simulink model "untitled"  (R2021b)
settings: Solver=VariableStepAuto  StartTime=0.0  StopTime=10.0  RelTol=1e-3
values from neighbouring files (symbols this model uses):
  simu = simulationClass()    [wecSimInputFile.m]
undefined symbols (not defined in the file or in its folder): DiscIntNeverNeededParam, PTOSimBlock
settings Model: Creator=jleonqu  LastModifiedBy=jleonqu

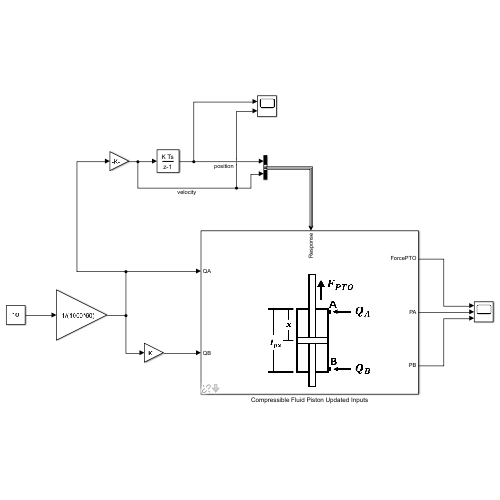
[thumbnail: Simulink's stored preview of the top-level diagram]
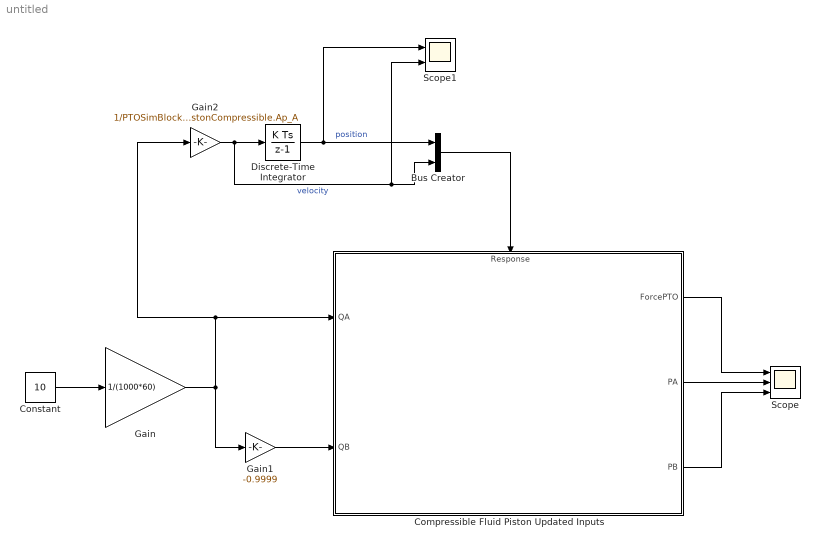
== system untitled ==
  Bus Creator : BusCreator  Inputs=2
  Compressible Fluid Piston Updated Inputs : Subsystem  AncestorBlock=PTOSim_Lib_UpdatedV3/Hydraulic/Compressible Fluid Piston Updated Inputs  mask{PTOSimBlock=PTOSimBlock(1), InputFileText=Use WEC-Sim input file to define PTO parameters, Ap_A=0, Ap_B=0, PistonStroke=0, BulkModulus=0, xi_piston=0, pAi=0, pBi=0}
      mask prompts: PTOSimBlock "Piston Name"; Ap_A "Piston area A [m]"; Ap_B "Piston area B [m]"; PistonStroke "Piston stroke [m]"; BulkModulus "Fluid Bulk Modulus [Pa]"; xi_piston "Piston initial displacement from A [m]"; pAi "Port A Initial pressure [Pa]"; pBi "Port B Initial pressure [Pa]"
      mask help:
      | PTO-Sim Compressible Fluid Piston
      |
      | This block simualtes a hydraulic cylinder using a compressible fluid model. The block inputs are Response, QA and QB. Response is the signal output of the block Rotational PTO Actuation Force. QA and QB are the flow rate for port A and port B of the cylinder. The outputs of the block are ForcePTO, PA, and PB.
      mask init:
      | if exist('PTOSimBlock','var')
      |     h=[gcb '/To Workspace'];
      |     responseName=['PTOSimBlock' num2str(PTOSimBlock.PTOSimBlockNum) '_out'];
      |     set_param(h,'VariableName',responseName);
      | end
      | clear h responseName
      | %HydraulicBlock.checkLoc('W');
      settings: PortSchema="{\"entries\":[{\"content\":{\"sides\":[{\"content\":{\"connectorIds\":[\"In1\",\"In2\"]},\"type\":\"ConnectorPlacement.EquallySpacedRectSide\",\"uuid\":\"572dbc7c-8f4c-46fc-9000-663c89355fbd\"},{\"content\":{\"connectorIds\":[\"Out1\",\"Out2\",\"Out3\"],\"side\":\"RIGHT\"},\"type\":\"ConnectorPlacement.EquallySpacedRectSide\",\"uuid\":\"3b7821ce-a540-4de1-8f34-0d55375c774c\"},{\"content\":{\"connectorIds\":[\"In3\"],\"side\":\"TOP\"},\"type\":\"ConnectorPlacement.EquallySpacedRectSide\",\"uuid\":\"b6f5c275-868d-447d-b609-cdda14e9f222\"},{\"content\":{\"connectorIds\":[],\"side\":\"HIDDEN\"},\"type\":\"ConnectorPlacement.EquallySpacedRectSide\",\"uuid\":\"5b34aa5d-01fb-4d75-9f22-3e4ce64ee132\"}]},\"type\":\"ConnectorPlacement.EquallySpacedConnector\",\"uuid\":\"5b16a2f7-6624-4a26-89bf-8d87cef610e1\"}],\"packageUris\":[\"http://schema.mathworks.com/mf0/Connector/R2020b\"],\"version\":\"1.0\"}"
      mask Help:
      | This block simualtes a hydraulic cylinder using a compressible fluid model. The block inputs are Response and HydraulicInput. Response is the signal output of the block Rotational PTO Actuation Force. HydraulicInput is a two signal vector with the information of the flow rate for port A and port B of the cylinder. The output of the block is PistonOutput, which is a three signal vector with PressureA, PressureB, and ForcePTO.
      | 
      | The outputs are calculated using the model presented in the following link: http://wec-sim.github.io/WEC-Sim/master/user/advanced_features.html#pto-sim
      mask DialogControl ParameterGroupVar Prompt: Custom Parameters
      mask DialogControl PistonProperties Prompt: Piston Properties
      mask DialogControl InitialConditions Prompt: Initial Conditions
      mask Display: image('DoubleActingPiston.png'); % Use "Edit Image" on toolstrip to change.
  Constant : Constant  Value=10
  Discrete-Time Integrator : DiscreteIntegrator  SampleTime=-1  ICPrevOutput=DiscIntNeverNeededParam  ICPrevScaledInput=DiscIntNeverNeededParam
  Gain : Gain  Gain=1/(1000*60)
  Gain1 : Gain  Gain=-0.9999
  Gain2 : Gain  Gain=1/PTOSimBlock(1).HydPistonCompressible.Ap_A
  Scope : Scope  NumInputPorts=3
  Scope1 : Scope  NumInputPorts=2
  wires:
  Constant/1 -> Gain/1
  Gain1/1 -> Compressible Fluid Piston Updated Inputs/2(QB)
  Gain/1 -> Gain1/1, Compressible Fluid Piston Updated Inputs/1(QA), Gain2/1
  Gain2/1 -> Scope1/2, Bus Creator/2, Discrete-Time Integrator/1  "velocity"
  Discrete-Time Integrator/1 -> Scope1/1, Bus Creator/1  "position"
  Bus Creator/1 -> Compressible Fluid Piston Updated Inputs/3(Response)
  Compressible Fluid Piston Updated Inputs/1(ForcePTO) -> Scope/1
  Compressible Fluid Piston Updated Inputs/2(PA) -> Scope/2
  Compressible Fluid Piston Updated Inputs/3(PB) -> Scope/3

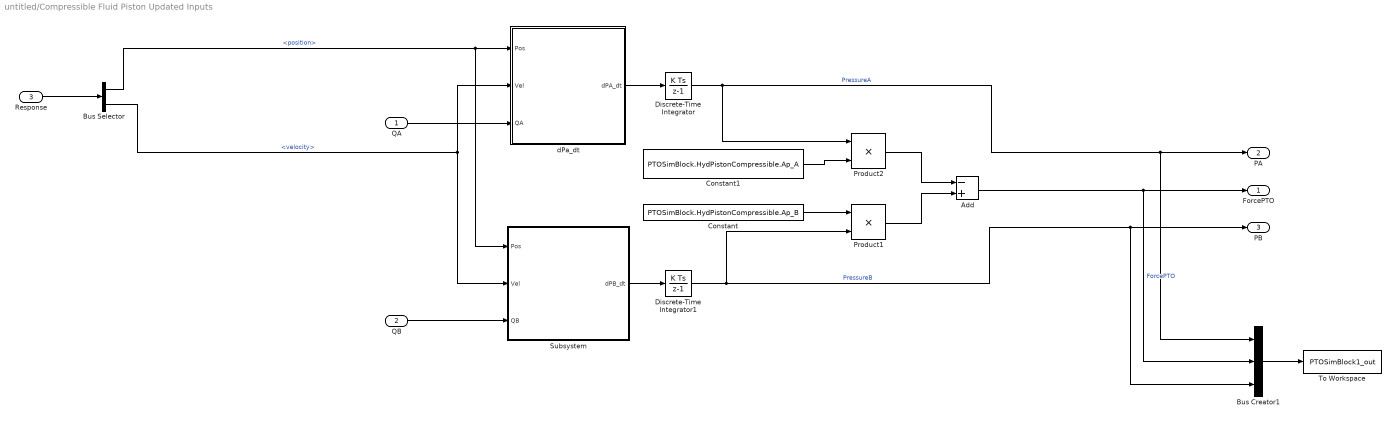
== system untitled/Compressible Fluid Piston Updated Inputs ==
  QA : Inport
  QB : Inport  Port=2
  Response : Inport  Port=3
  Add : Sum  Inputs=-+
  Bus Creator1 : BusCreator  Inputs=3
  Bus Selector : BusSelector  OutputSignals=position,velocity
  Constant : Constant  Value=PTOSimBlock.HydPistonCompressible.Ap_B
  Constant1 : Constant  Value=PTOSimBlock.HydPistonCompressible.Ap_A
  Discrete-Time Integrator : DiscreteIntegrator  InitialCondition=PTOSimBlock.HydPistonCompressible.pAi  SampleTime=-1  ICPrevOutput=DiscIntNeverNeededParam  ICPrevScaledInput=DiscIntNeverNeededParam
  Discrete-Time Integrator1 : DiscreteIntegrator  InitialCondition=PTOSimBlock.HydPistonCompressible.pBi  SampleTime=-1  ICPrevOutput=DiscIntNeverNeededParam  ICPrevScaledInput=DiscIntNeverNeededParam
  Product1 : Product
  Product2 : Product
  Subsystem : Subsystem  AncestorBlock=PTOSim_Lib_UpdatedV3/Hydraulic/Compressible Fluid Piston Updated/Subsystem
  To Workspace : ToWorkspace  VariableName=PTOSimBlock1_out  SaveFormat=Structure With Time  SampleTime=simu.dtOut
  dPa_dt : Subsystem  AncestorBlock=PTOSim_Lib_UpdatedV3/Hydraulic/Compressible Fluid Piston Updated/dPa_dt
  ForcePTO : Outport
  PA : Outport  Port=2
  PB : Outport  Port=3
  wires:
  Bus Selector/1 -> dPa_dt/1(Pos), Subsystem/1(Pos)  "<position>"
  Discrete-Time Integrator/1 -> Product2/1, Bus Creator1/1, PA/1  "PressureA"
  Response/1 -> Bus Selector/1
  Subsystem/1(dPB_dt) -> Discrete-Time Integrator1/1
  Bus Selector/2 -> dPa_dt/2(Vel), Subsystem/2(Vel)  "<velocity>"
  Constant/1 -> Product1/1
  Product2/1 -> Add/1
  dPa_dt/1(dPA_dt) -> Discrete-Time Integrator/1
  Product1/1 -> Add/2
  QB/1 -> Subsystem/3(QB)
  Bus Creator1/1 -> To Workspace/1
  Add/1 -> ForcePTO/1, Bus Creator1/2  "ForcePTO"
  Discrete-Time Integrator1/1 -> Product1/2, PB/1, Bus Creator1/3  "PressureB"
  Constant1/1 -> Product2/2
  QA/1 -> dPa_dt/3(QA)

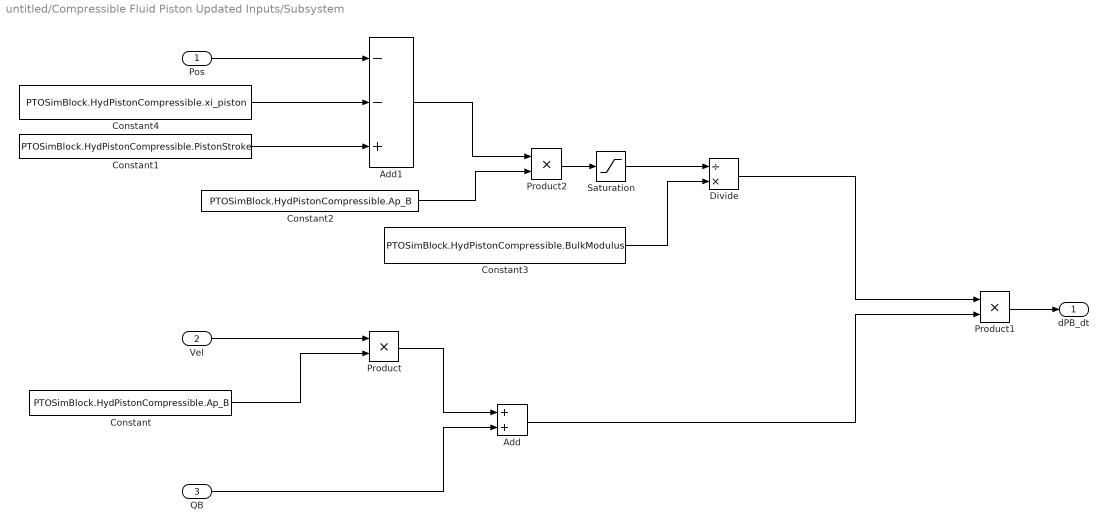
== system untitled/Compressible Fluid Piston Updated Inputs/Subsystem ==
  Pos : Inport
  Vel : Inport  Port=2
  QB : Inport  Port=3
  Add : Sum
  Add1 : Sum  Inputs=--+
  Constant : Constant  Value=PTOSimBlock.HydPistonCompressible.Ap_B
  Constant1 : Constant  Value=PTOSimBlock.HydPistonCompressible.PistonStroke
  Constant2 : Constant  Value=PTOSimBlock.HydPistonCompressible.Ap_B
  Constant3 : Constant  Value=PTOSimBlock.HydPistonCompressible.BulkModulus
  Constant4 : Constant  Value=PTOSimBlock.HydPistonCompressible.xi_piston
  Divide : Product  Inputs=/*
  Product : Product
  Product1 : Product
  Product2 : Product
  Saturation : Saturate  UpperLimit=inf  LowerLimit=1e-10
  dPB_dt : Outport
  wires:
  Constant4/1 -> Add1/2
  Constant1/1 -> Add1/3
  Product1/1 -> dPB_dt/1
  Divide/1 -> Product1/1
  Constant3/1 -> Divide/2
  Product2/1 -> Saturation/1
  Constant2/1 -> Product2/2
  Add1/1 -> Product2/1
  Pos/1 -> Add1/1
  Add/1 -> Product1/2
  QB/1 -> Add/2
  Product/1 -> Add/1
  Constant/1 -> Product/2
  Vel/1 -> Product/1
  Saturation/1 -> Divide/1

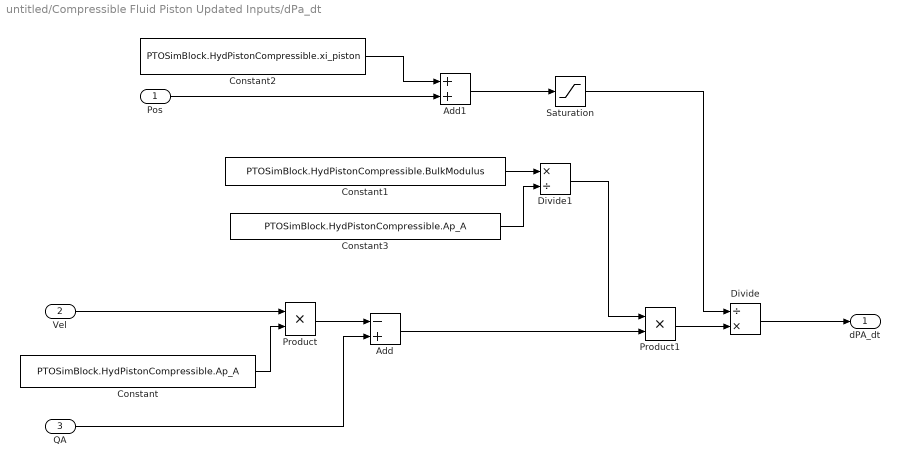
== system untitled/Compressible Fluid Piston Updated Inputs/dPa_dt ==
  Pos : Inport
  Vel : Inport  Port=2
  QA : Inport  Port=3
  Add : Sum  Inputs=-+
  Add1 : Sum
  Constant : Constant  Value=PTOSimBlock.HydPistonCompressible.Ap_A
  Constant1 : Constant  Value=PTOSimBlock.HydPistonCompressible.BulkModulus
  Constant2 : Constant  Value=PTOSimBlock.HydPistonCompressible.xi_piston
  Constant3 : Constant  Value=PTOSimBlock.HydPistonCompressible.Ap_A
  Divide : Product  Inputs=/*
  Divide1 : Product  Inputs=*/
  Product : Product
  Product1 : Product
  Saturation : Saturate  UpperLimit=inf  LowerLimit=1e-10
  dPA_dt : Outport
  wires:
  Add1/1 -> Saturation/1
  Constant2/1 -> Add1/1
  Pos/1 -> Add1/2
  Product/1 -> Add/1
  QA/1 -> Add/2
  Constant/1 -> Product/2
  Add/1 -> Product1/2
  Divide/1 -> dPA_dt/1
  Product1/1 -> Divide/2
  Vel/1 -> Product/1
  Saturation/1 -> Divide/1
  Constant1/1 -> Divide1/1
  Constant3/1 -> Divide1/2
  Divide1/1 -> Product1/1
